simulink model "Three_ph_AC_Volt_Controller"  (R2024b)
settings: Solver=VariableStepAuto  StartTime=0.0  StopTime=1  RelTol=1e-3
libraries: spsThyristorLib x6, spsVoltageMeasurementLib x6, spsACVoltageSourceLib x3, spsGroundLib x3, spsSeriesRLCBranchLib x3, spsRMSLib x1, sps_lib x1
settings Model: Creator=hp  LastModifiedBy=hp

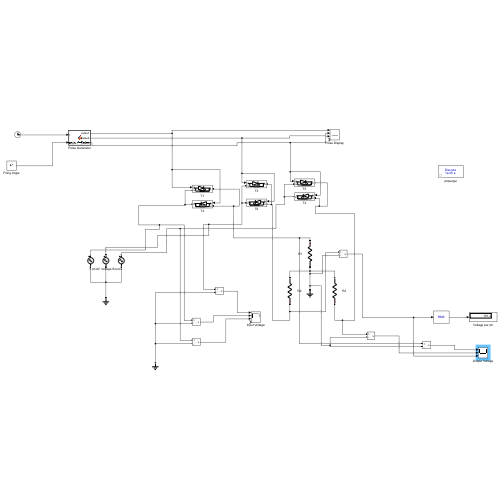
[thumbnail: Simulink's stored preview of the top-level diagram]
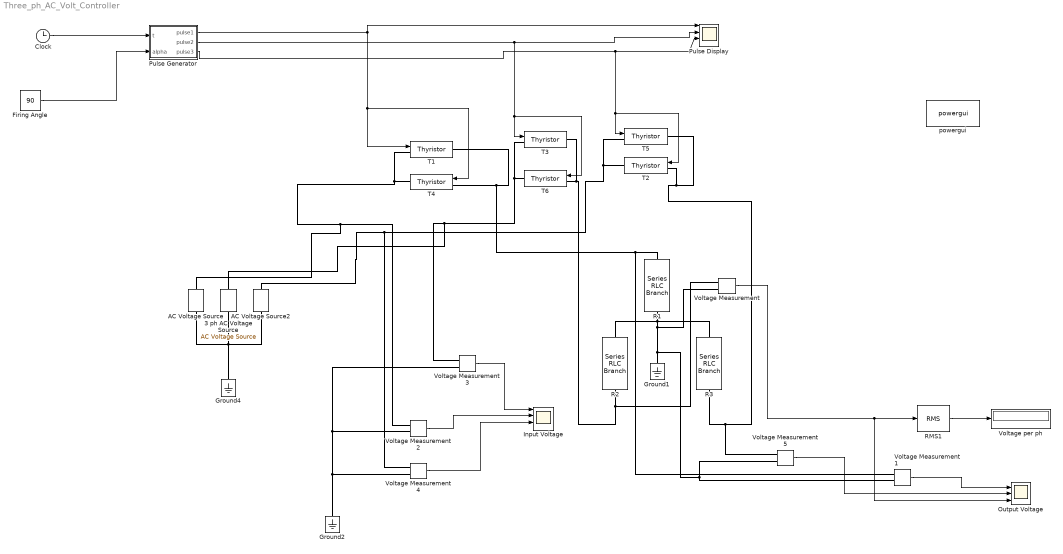
== system Three_ph_AC_Volt_Controller ==
  3 ph AC Voltage Source : spsACVoltageSourceLib/AC Voltage Source  Amplitude=311  Phase=-120  Frequency=50  SampleTime=0  Measurements=None  BusType=swing  Pref=10e3  Qref=0  Qmin=-inf  Qmax=+inf
  AC Voltage Source : spsACVoltageSourceLib/AC Voltage Source  Amplitude=311  Phase=0  Frequency=50  SampleTime=0  Measurements=None  BusType=swing  Pref=10e3  Qref=0  Qmin=-inf  Qmax=+inf
  AC Voltage Source2 : spsACVoltageSourceLib/AC Voltage Source  Amplitude=311  Phase=120  Frequency=50  SampleTime=0  Measurements=None  BusType=swing  Pref=10e3  Qref=0  Qmin=-inf  Qmax=+inf
  Clock : Clock
  Firing Angle : Constant  Value=90
  Ground1 : spsGroundLib/Ground  LConnTagsString=a
  Ground2 : spsGroundLib/Ground  LConnTagsString=a
  Ground4 : spsGroundLib/Ground  LConnTagsString=a
  Input Voltage : Scope  NumInputPorts=4
  Output Voltage : Scope  NumInputPorts=3
  Pulse Display : Scope  NumInputPorts=4
  Pulse Generator : MATLAB Function  TreatAsAtomicUnit=on
  R1 : spsSeriesRLCBranchLib/Series RLC Branch  LConnTagsString=__new0  RConnTagsString=__new0  BranchType=R  Resistance=10000  Inductance=1e-3  SetiL0=off  InitialCurrent=0  Capacitance=1e-6  Setx0=off  InitialVoltage=0  Measurements=None
  R2 : spsSeriesRLCBranchLib/Series RLC Branch  LConnTagsString=__new0  RConnTagsString=__new0  BranchType=R  Resistance=10000  Inductance=1e-3  SetiL0=off  InitialCurrent=0  Capacitance=1e-6  Setx0=off  InitialVoltage=0  Measurements=None
  R3 : spsSeriesRLCBranchLib/Series RLC Branch  LConnTagsString=__new0  RConnTagsString=__new0  BranchType=R  Resistance=10000  Inductance=1e-3  SetiL0=off  InitialCurrent=0  Capacitance=1e-6  Setx0=off  InitialVoltage=0  Measurements=None
  RMS1 : spsRMSLib/RMS  TrueRMS=on  Freq=60  RMSInit=120  Ts=0
  T{1..6} (6 alike) : spsThyristorLib/Thyristor  Ron=0.001  Lon=0  Vf=0.8  IC=0  Rs=1000  Cs=1*1e-9  Measurements=off
  Voltage Measurement{,1..5} (6 alike) : spsVoltageMeasurementLib/Voltage Measurement  PhasorSimulation=off  OutputType=Complex  PSBequivalent=0
  Voltage per ph : Display
  powergui : sps_lib/powergui  Priority=1  SimulationMode=Discrete  SampleTime=1e-5  frequency=60  Iterations=50  frequencyindice=50  Pbase=100e6  ErrMax=1e-4  UnitsV=kV  UnitsW=MW  buscounter=0  FunctionMessages=off  echomessages=off  EnableUseOfTLC=off  CurrentSourceSwitches=off  DisableSnubberDevices=off  DisableRonSwitches=off  DisableVfSwitches=off  DisplayEquations=off  AutomaticDiscreteSolvers=off  SolverType=Tustin/Backward Euler (TBE)  Interpol=off  ExternalGateDelay=off  methode=off  Ts=100  x0status=blocks  SPID=on  SwTol=0  HookPort=off  NonlinearTolerance=1e-4  nMaxIteration=100  ContinueOnMaxIteration=off  RestoreLinks=warning  ResistiveCurrentMeasurement=off  Frange=[0:2:500]  Ylog=off  Xlog=on  ShowGrid=off  save=off  variable=ZData  structure=0  ZoomFFT=off  StartTime=0.0  cycles=1  DisplayStyle=1  fundamental=60  FreqAxis=off  MaxFrequency=1000  frequencyindicesteady=1  RmsSteady=1  display=off
  wires:
  Voltage Measurement/1 -> Output Voltage/3, RMS1/1
  RMS1/1 -> Voltage per ph/1
  Firing Angle/1 -> Pulse Generator/2(alpha)
  Voltage Measurement1/1 -> Output Voltage/1
  Voltage Measurement5/1 -> Output Voltage/2
  Voltage Measurement4/1 -> Input Voltage/3
  Voltage Measurement2/1 -> Input Voltage/2
  Voltage Measurement3/1 -> Input Voltage/1
  Clock/1 -> Pulse Generator/1(t)
  Pulse Generator/1(pulse1) -> Pulse Display/1, T4/1, T1/1
  Pulse Generator/2(pulse2) -> Pulse Display/2, T6/1, T3/1
  Pulse Generator/3(pulse3) -> T2/1, T5/1, Pulse Display/3
  connections:
  T4/LConn1 -- T1/RConn1 -- Voltage Measurement1/LConn1 -- R1/LConn1
  T3/RConn1 -- Voltage Measurement/LConn1 -- R2/LConn1 -- T6/LConn1
  T5/RConn1 -- Voltage Measurement5/LConn1 -- R3/LConn1 -- T2/LConn1
  T3/LConn1 -- Voltage Measurement3/LConn1 -- 3 ph AC Voltage Source/RConn1 -- T6/RConn1
  T5/LConn1 -- AC Voltage Source2/RConn1 -- Voltage Measurement4/LConn1 -- T2/RConn1
  R2/RConn1 -- Voltage Measurement5/LConn2 -- Voltage Measurement1/LConn2 -- Ground1/LConn1 -- Voltage Measurement/LConn2 -- R3/RConn1 -- R1/RConn1
  Voltage Measurement2/LConn2 -- Ground2/LConn1 -- Voltage Measurement4/LConn2 -- Voltage Measurement3/LConn2
  T1/LConn1 -- Voltage Measurement2/LConn1 -- AC Voltage Source/RConn1 -- T4/RConn1
  AC Voltage Source2/LConn1 -- Ground4/LConn1 -- AC Voltage Source/LConn1 -- 3 ph AC Voltage Source/LConn1

== matlab function Three_ph_AC_Volt_Controller/Pulse Generator ==
  data: t input; pulse1 output; alpha input; pulse2 output; pulse3 output
function [pulse1, pulse2, pulse3] = generatePulses(t, alpha)
% Inputs:
%   t     - simulation time (from Simulink clock)
%   alpha - firing angle in degrees (0 to 180 typically)
% Outputs:
%   pulse1, pulse2, pulse3 - three output pulses (0 or 1)

% Constants
f = 100;                  % Frequency in Hz
T = 1 / f;                % Period in seconds
alpha_time = (alpha / 360) *0.02;  % Convert firing angle to time delay

% Pulse width (adjustable)
pulse_width = 0.0010;     % 500 µs wide pulse

% Time in current cycle
t_mod = mod(t, T);

% Pulse start times (120° = T/3 apart)
start1 = alpha_time;
start2 = mod(alpha_time + 2*T/3, T);   % +120°
start3 = mod(alpha_time + T/3, T); % +240°

% Generate pulses
pulse1 = double(t_mod >= start1-pulse_width/2 && t_mod < start1 + pulse_width/2);
pulse2 = double(t_mod >= start2-pulse_width/2 && t_mod < start2 + pulse_width/2);
pulse3 = double(t_mod >= start3-pulse_width/2 && t_mod < start3 + pulse_width/2);
